simulink model "DriveTrain_Modular1"  (R2019a)
settings: Solver=FixedStepAuto  StartTime=0.0  StopTime=0.6  FixedStep=Ts  RelTol=1e-3
InitFcn:
  | DriveTrainInitialise;
undefined symbols (not defined in the file or in its folder): C, D, fsw, KdAW, KdI, KdP, KqAW, KqI, KqP, Ld, Lq, PM, Pmax, PolePairs, RotorInertia, Rs, Tmax, Ts, Tsc, Vnom
libraries: fl_lib x25, nesl_utility x13, ee_lib x5, eeGeneralControl x2, eePmsmFieldOrientedControl x1
settings Model: OrderedModelArguments=off  Creator=plewi  LastModifiedBy=plewi
settings SolverCC: ZeroCrossAlgorithm=Adaptive
settings DataIOCC: OutputOption=SpecifiedOutputTimes  OutputTimes=SDO_OutputTimes  ReturnWorkspaceOutputsName=SDOSimTest_Log
settings DebuggingCC: IgnoredZcDiagnostic=none

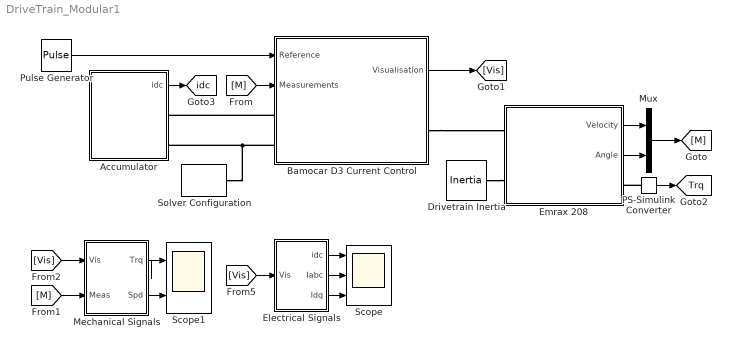
== system DriveTrain_Modular1 ==
  Accumulator : Subsystem  AncestorBlock=AccumulatorLIB/Accumulator (Simple)
  Bamocar D3 Current Control : Subsystem  AncestorBlock=InverterLIB/Bamocar D3 Current Control (Simple IGBTs)  mask(Bamocar D3 Current Controlled (Simple Diode)){Vnom=Vnom, Pmax=Pmax, Tmax=Tmax, Iq_max=800, p=PolePairs, Vdc_on=20, Ts=Ts, Tsc=Tsc, Ron=0.01, Goff=1e-8, Vf=0.5, diode_Vf=1.55, diode_Ron=0.01, diode_Goff=1e-8, RefType=Zero d-axis control, psim=PM, AxisAlignment=Q-axis, Kp_id=KdP, Ki_id=KdI, Kaw_id=KdAW, Kp_iq=KqP, Ki_iq=KqI, Kaw_iq=KqAW, AxisPrio=D-axis, CPWMMode=SVM: space vector modulation, SamplingMode=Natural, fsw=fsw}
      mask prompts: Vnom "Nominal dc-link voltage (V):"; Pmax "Maximum power (W):"; Tmax "Maximum torque (N*m):"; Iq_max "Maximum current, Iq (A):"; p "Number of rotor pole pairs:"; Vdc_on "Inverter dc-link voltage threshold (V):"; Ts "Fundamental sample time (s):"; Tsc "Control sample time (s):"; Ron "On-state resistance (Ohm):"; Goff "Off-state conductance (Siemens):"; Vf "Switching Threshold:"; diode_Vf "Forward voltage (V):"; diode_Ron "On resistance (Ohm):"; diode_Goff "Off conductance (Siemens):"; RefType "Current references:"; psim "Permanent magnet flux linkage (Wb):"; AxisAlignment "Phase-a axis alignment:"; Kp_id "D-axis current proportional gain:"; Ki_id "D-axis current integral gain:"; Kaw_id "D-axis current anti-windup gain:"; Kp_iq "Q-axis current proportional gain:"; Ki_iq "Q-axis current integral gain:"; Kaw_iq "Q-axis current anti-windup gain:"; AxisPrio "Axis prioritization:"; CPWMMode "PWM method:"; SamplingMode "Sampling mode:"; fsw "Switching frequency (Hz):"
      mask help: This block implements a PMSM field-oriented control structure, similar to the Bamocar D3. It operates under current/torque control.
      mask Help: web(nesl_help(gcbh))
      mask TypeOptions Vnom:
      | Inverter Controller/PMSM Field-Oriented
      | Control/Vnom
      mask TypeOptions Pmax:
      | Inverter Controller/PMSM Field-Oriented
      | Control/Pmax
      mask TypeOptions Tmax:
      | Inverter Controller/PMSM Field-Oriented
      | Control/Tmax
      mask TypeOptions p:
      | Inverter Controller/PMSM Field-Oriented
      | Control/p
      mask TypeOptions Vdc_on:
      | Inverter Controller/PMSM Field-Oriented
      | Control/Vdc_on
      mask TypeOptions Ts:
      | Inverter Controller/PMSM Field-Oriented
      | Control/Ts
      mask TypeOptions Tsc:
      | Inverter Controller/PMSM Field-Oriented
      | Control/Tsc
      mask TypeOptions Ron:
      | Three-Phase
      | Inverter/Switch/R_closed | Three-Phase
      | Inverter/Switch1/R_closed | Three-Phase
      | Inverter/Switch2/R_closed | Three-Phase
      | Inverter/Switch3/R_closed | Three-Phase
      | Inverter/Switch4/R_closed | Three-Phase
      | Inverter/Switch5/R_closed
      mask TypeOptions Goff:
      | Three-Phase
      | Inverter/Switch/G_open | Three-Phase
      | Inverter/Switch1/G_open | Three-Phase
      | Inverter/Switch2/G_open | Three-Phase
      | Inverter/Switch3/G_open | Three-Phase
      | Inverter/Switch4/G_open | Three-Phase
      | Inverter/Switch5/G_open
      mask TypeOptions Vf:
      | Three-Phase
      | Inverter/Switch/Threshold | Three-Phase
      | Inverter/Switch1/Threshold | Three-Phase
      | Inverter/Switch2/Threshold | Three-Phase
      | Inverter/Switch3/Threshold | Three-Phase
      | Inverter/Switch4/Threshold | Three-Phase
      | Inverter/Switch5/Threshold
      mask TypeOptions diode_Vf:
      | Three-Phase
      | Inverter/Diode1/Vf | Three-Phase
      | Inverter/Diode2/Vf | Three-Phase
      | Inverter/Diode3/Vf | Three-Phase
      | Inverter/Diode4/Vf | Three-Phase
      | Inverter/Diode5/Vf | Three-Phase
      | Inverter/Diode6/Vf
      mask TypeOptions diode_Ron:
      | Three-Phase
      | Inverter/Diode1/Ron | Three-Phase
      | Inverter/Diode2/Ron | Three-Phase
      | Inverter/Diode3/Ron | Three-Phase
      | Inverter/Diode4/Ron | Three-Phase
      | Inverter/Diode5/Ron | Three-Phase
      | Inverter/Diode6/Ron
      mask TypeOptions diode_Goff:
      | Three-Phase
      | Inverter/Diode1/Goff | Three-Phase
      | Inverter/Diode2/Goff | Three-Phase
      | Inverter/Diode3/Goff | Three-Phase
      | Inverter/Diode4/Goff | Three-Phase
      | Inverter/Diode5/Goff | Three-Phase
      | Inverter/Diode6/Goff
      mask TypeOptions RefType:
      | Inverter Controller/PMSM Field-Oriented
      | Control/RefType
      mask TypeOptions psim:
      | Inverter Controller/PMSM Field-Oriented
      | Control/psim
      mask TypeOptions AxisAlignment:
      | Inverter Controller/PMSM Field-Oriented
      | Control/AxisAlignment
      mask TypeOptions Kp_id:
      | Inverter Controller/PMSM Field-Oriented
      | Control/Kp_id
      mask TypeOptions Ki_id:
      | Inverter Controller/PMSM Field-Oriented
      | Control/Ki_id
      mask TypeOptions Kaw_id:
      | Inverter Controller/PMSM Field-Oriented
      | Control/Kaw_id
      mask TypeOptions Kp_iq:
      | Inverter Controller/PMSM Field-Oriented
      | Control/Kp_iq
      mask TypeOptions Ki_iq:
      | Inverter Controller/PMSM Field-Oriented
      | Control/Ki_iq
      mask TypeOptions Kaw_iq:
      | Inverter Controller/PMSM Field-Oriented
      | Control/Kaw_iq
      mask TypeOptions AxisPrio:
      | Inverter Controller/PMSM Field-Oriented
      | Control/AxisPrio
      mask TypeOptions CPWMMode:
      | Inverter Controller/PMSM Field-Oriented
      | Control/CPWMMode
      mask TypeOptions SamplingMode:
      | Inverter Controller/PMSM Field-Oriented
      | Control/SamplingMode
      mask TypeOptions fsw:
      | Inverter Controller/PMSM Field-Oriented
      | Control/fsw
      mask DialogControl Container4 Prompt: General
      mask DialogControl Container11 Prompt: Electrical
      mask DialogControl Container12 Prompt: Capacitor Bank
      mask DialogControl Container16 Prompt: IGBTs
      mask DialogControl Container17 Prompt: Protection Diodes
      mask DialogControl Container5 Prompt: Outer Loop
      mask DialogControl Container6 Prompt: Inner Loop
      mask DialogControl Container7 Prompt: PWM
      mask Display: image('C:\Users\plewi\Documents\University\6-Sixth Year\MUR\MUR-E_Simulation_2019\Images\bamocar_d3.PNG');
  Drivetrain Inertia : fl_lib/Mechanical/Rotational Elements/Inertia  inertia=J kg*m^2  w_specify=off  w_priority=High  w=0 rad/s  w_nominal_specify=off  w_nominal_unit=rad/s  w_nominal_value=1  t_specify=off  t_priority=None  t=0 N*m  t_nominal_specify=off  t_nominal_unit=N*m  t_nominal_value=1
  Electrical Signals : Subsystem
  Emrax 208 : Subsystem  AncestorBlock=MotorLIB/Emrax 208  mask(Emrax 208){nPolePairs=PolePairs, pm_flux_linkage=PM, Ld=Ld, Lq=Lq, L0=0, Rs=Rs, zero_sequence=ee.enum.park.zerosequence.exclude, J=RotorInertia}
      mask prompts: nPolePairs "Number of pole pairs"; pm_flux_linkage "Permanent magnet flux linkage"; Ld "Stator d-axis inductance, Ld"; Lq "Stator q-axis inductance, Lq"; L0 "Stator zero-sequence inductance, L0"; Rs "Stator resistance per phase, Rs"; zero_sequence "Zero sequence"; J "Rotor inertia (g cm^2)"
      mask TypeOptions nPolePairs:
      | Permanent Magnet
      | Synchronous Motor/nPolePairs
      mask TypeOptions pm_flux_linkage:
      | Permanent Magnet
      | Synchronous Motor/pm_flux_linkage
      mask TypeOptions Ld:
      | Permanent Magnet
      | Synchronous Motor/Ld
      mask TypeOptions Lq:
      | Permanent Magnet
      | Synchronous Motor/Lq
      mask TypeOptions L0:
      | Permanent Magnet
      | Synchronous Motor/L0
      mask TypeOptions Rs:
      | Permanent Magnet
      | Synchronous Motor/Rs
      mask TypeOptions zero_sequence:
      | Permanent Magnet
      | Synchronous Motor/zero_sequence
      mask TypeOptions J:
      | Permanent Magnet
      | Synchronous Motor/J
      mask DialogControl Container4 Prompt: Main
  Mechanical Signals : Subsystem
  Mux : Mux  Inputs=2
  PS-Simulink Converter : nesl_utility/PS-Simulink Converter  PhysicalDomain=network_engine_domain  SubClassName=ps_output  LeftPortType=input  RightPortType=output  PseudoPeriodic=off  Frequencies=[]  Unit=1  AffineConversion=off
  Pulse Generator : DiscretePulseGenerator  PulseType=Time based  Amplitude=5  Period=0.6  PulseWidth=50  PhaseDelay=0.05
  Scope : Scope  NumInputPorts=3
  Scope1 : Scope  NumInputPorts=2
  Solver Configuration : nesl_utility/Solver Configuration  PhysicalDomain=network_engine_domain  SubClassName=solver  LeftPortType=input  RightPortType=generic  Tones=[]  Harmonics=[]  SimulateNoise=off  Profile=off  UseLocalSampling=off  EnableSwitchedLinearOptims=on  FrequencyDomain=off  UseCCode=off  RelTol=0.001  AbsTol=1e-06  MinStep=1e-09  ToWorkspace=off  RevertToSquareIcSolve=off  NumHomotopyIterations=100  PhasorMode=off  PhasorModeNumHarmonics=1  DoDC=off  ResidualTolerance=1e-09  UseLocalSolver=off  LocalSolverChoice=NE_BACKWARD_EULER_ADVANCER  LocalSolverSampleTime=0.001  DoFixedCost=off  MaxNonlinIter=3  MaxModeIter=2  LinearAlgebra=auto  EquationFormulation=NE_TIME_EF  DelaysMemoryBudget=1024  AutomaticFiltering=on  FilteringTimeConstant=0.001  PartitionStorageMethod=AS_NEEDED  PartitionMemoryBudget=1024  PartitionMethod=ROBUST
  tag scope: Trq=global, idc=global
  wires:
  Mux/1 -> [M]
  [M] -> Bamocar D3 Current Control/2(Measurements)
  Emrax 208/1(Velocity) -> Mux/1
  Emrax 208/2(Angle) -> Mux/2
  Bamocar D3 Current Control/1(Visualisation) -> [Vis]
  PS-Simulink Converter/1 -> [Trq]
  Accumulator/1(idc) -> [idc]
  Electrical Signals/1(idc) -> Scope/1
  Electrical Signals/3(Idq) -> Scope/3
  [M] -> Mechanical Signals/2("Meas ")
  [Vis] -> Mechanical Signals/1(Vis)
  Electrical Signals/2(Iabc) -> Scope/2
  Mechanical Signals/1(Trq) -> Scope1/1
  Mechanical Signals/2(Spd) -> Scope1/2
  [Vis] -> Electrical Signals/1(Vis)
  Pulse Generator/1 -> Bamocar D3 Current Control/1(Reference)
  connections:
  Bamocar D3 Current Control/LConn2 -- Solver Configuration/RConn1 -- Accumulator/RConn2
  PS-Simulink Converter/LConn1 -- Emrax 208/RConn1
  Bamocar D3 Current Control/LConn1 -- Accumulator/RConn1
  Bamocar D3 Current Control/RConn1 -- Emrax 208/LConn1
  Drivetrain Inertia/LConn1 -- Emrax 208/LConn2

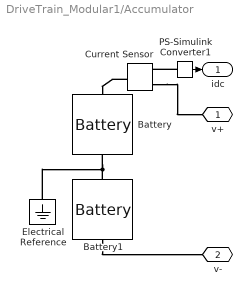
== system DriveTrain_Modular1/Accumulator ==
  Battery : ee_lib/Sources/Battery  Vnom=Vnom/2 V  R1=0.001 Ohm  prm_AH=1  AH=14000 hr*A  V1=470 V  AH1=5000 hr*A  prm_R2=1  R2=inf Ohm  prm_dyn=1  Rp1=0.005 Ohm  tau1=30 s  Rp2=0.005 Ohm  tau2=30 s  Rp3=0.005 Ohm  tau3=30 s  Rp4=0.005 Ohm  tau4=30 s  Rp5=0.005 Ohm  tau5=30 s  prm_fade=1  N_fade=100  AH_fade=45 hr*A  R1_fade=2.02 Ohm  V1_fade=10.35 V  i_specify=off  i_priority=Low  i=0 A  i_nominal_specify=off  i_nominal_unit=A  i_nominal_value=1  v_specify=on  v_priority=High  v=Vnom/2 V  v_nominal_specify=off  v_nominal_unit=V  v_nominal_value=1  charge_specify=on  charge_priority=None  charge=7000 hr*A  charge_nominal_specify=off  charge_nominal_unit=hr*A  charge_nominal_value=1  num_cycles_specify=on  num_cycles_priority=None  num_cycles=0  num_cycles_nominal_specify=off  num_cycles_nominal_unit=1  num_cycles_nominal_value=1  thermal_mass=30000 J/K  Tmeas=298.15 K  Vnom_T2=12 V  R1_T2=2.2 Ohm  V1_T2=11.4 V  R2_T2=2200 Ohm  Rp1_T2=0.005 Ohm  tau1_T2=30 s  Rp2_T2=0.005 Ohm  tau2_T2=30 s  Rp3_T2=0.005 Ohm  tau3_T2=30 s  Rp4_T2=0.005 Ohm  tau4_T2=30 s  Rp5_T2=0.005 Ohm  tau5_T2=30 s  Tmeas2=273.15 K  temperature_specify=off  temperature_priority=High  temperature=298.15 K  temperature_nominal_specify=off  temperature_nominal_unit=K  temperature_nominal_value=1
      settings: SourceProductName=Simscape Electrical
  Battery1 : ee_lib/Sources/Battery  Vnom=Vnom/2 V  R1=0.001 Ohm  prm_AH=1  AH=14000 hr*A  V1=470 V  AH1=5000 hr*A  prm_R2=1  R2=inf Ohm  prm_dyn=1  Rp1=0.005 Ohm  tau1=30 s  Rp2=0.005 Ohm  tau2=30 s  Rp3=0.005 Ohm  tau3=30 s  Rp4=0.005 Ohm  tau4=30 s  Rp5=0.005 Ohm  tau5=30 s  prm_fade=1  N_fade=100  AH_fade=45 hr*A  R1_fade=2.02 Ohm  V1_fade=10.35 V  i_specify=off  i_priority=Low  i=0 A  i_nominal_specify=off  i_nominal_unit=A  i_nominal_value=1  v_specify=on  v_priority=High  v=Vnom/2 V  v_nominal_specify=off  v_nominal_unit=V  v_nominal_value=1  charge_specify=on  charge_priority=None  charge=7000 hr*A  charge_nominal_specify=off  charge_nominal_unit=hr*A  charge_nominal_value=1  num_cycles_specify=on  num_cycles_priority=None  num_cycles=0  num_cycles_nominal_specify=off  num_cycles_nominal_unit=1  num_cycles_nominal_value=1  thermal_mass=30000 J/K  Tmeas=298.15 K  Vnom_T2=12 V  R1_T2=2.2 Ohm  V1_T2=11.4 V  R2_T2=2200 Ohm  Rp1_T2=0.005 Ohm  tau1_T2=30 s  Rp2_T2=0.005 Ohm  tau2_T2=30 s  Rp3_T2=0.005 Ohm  tau3_T2=30 s  Rp4_T2=0.005 Ohm  tau4_T2=30 s  Rp5_T2=0.005 Ohm  tau5_T2=30 s  Tmeas2=273.15 K  temperature_specify=off  temperature_priority=High  temperature=298.15 K  temperature_nominal_specify=off  temperature_nominal_unit=K  temperature_nominal_value=1
      settings: SourceProductName=Simscape Electrical
  Current Sensor : fl_lib/Electrical/Electrical Sensors/Current Sensor
  Electrical Reference : fl_lib/Electrical/Electrical Elements/Electrical Reference
      settings: SourceProductName=Foundation Library
  PS-Simulink Converter1 : nesl_utility/PS-Simulink Converter  PhysicalDomain=network_engine_domain  SubClassName=ps_output  LeftPortType=input  RightPortType=output  PseudoPeriodic=off  Frequencies=[]  Unit=1  AffineConversion=off
  v+ : PMIOPort  Side=Right
  v- : PMIOPort  Port=2  Side=Right
  idc : Outport
  wires:
  PS-Simulink Converter1/1 -> idc/1
  connections:
  Battery1/RConn1 -- v-/RConn1
  PS-Simulink Converter1/LConn1 -- Current Sensor/RConn1
  Current Sensor/RConn2 -- v+/RConn1
  Current Sensor/LConn1 -- Battery/LConn1
  Battery1/LConn1 -- Electrical Reference/LConn1 -- Battery/RConn1

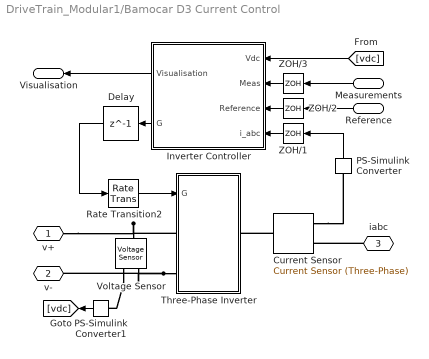
== system DriveTrain_Modular1/Bamocar D3 Current Control ==
  Reference : Inport
  Measurements : Inport  Port=2
  Current Sensor : ee_lib/Sensors & Transducers/Current Sensor (Three-Phase)
      settings: SourceProductName=Simscape Electrical
  Delay : Delay  DelayLength=1
  Inverter Controller : Subsystem
  PS-Simulink Converter : nesl_utility/PS-Simulink Converter  PhysicalDomain=network_engine_domain  SubClassName=ps_output  LeftPortType=input  RightPortType=output  PseudoPeriodic=off  Frequencies=[]  Unit=1  AffineConversion=off
  PS-Simulink Converter1 : nesl_utility/PS-Simulink Converter  PhysicalDomain=network_engine_domain  SubClassName=ps_output  LeftPortType=input  RightPortType=output  PseudoPeriodic=off  Frequencies=[]  Unit=1  AffineConversion=off
  Rate Transition2 : RateTransition  OutPortSampleTime=Ts
  Three-Phase Inverter : Subsystem
  Voltage Sensor : fl_lib/Electrical/Electrical Sensors/Voltage Sensor
  ZOH/1 : ZeroOrderHold  SampleTime=Tsc
  ZOH/2 : ZeroOrderHold  SampleTime=Tsc
  ZOH/3 : ZeroOrderHold  SampleTime=Tsc
  v+ : PMIOPort  Side=Left
  v- : PMIOPort  Port=2  Side=Left
  iabc : PMIOPort  Port=3  Side=Right
  Visualisation : Outport
  wires:
  Measurements/1 -> ZOH/3/1
  Delay/1 -> Rate Transition2/1
  Inverter Controller/2(G) -> Delay/1
  ZOH/1/1 -> Inverter Controller/4(i_abc)
  PS-Simulink Converter/1 -> ZOH/1/1
  ZOH/2/1 -> Inverter Controller/3(Reference)
  Rate Transition2/1 -> Three-Phase Inverter/1(G)
  Inverter Controller/1(Visualisation) -> Visualisation/1
  PS-Simulink Converter1/1 -> [vdc]
  [vdc] -> Inverter Controller/1(Vdc)
  ZOH/3/1 -> Inverter Controller/2(Meas)
  Reference/1 -> ZOH/2/1
  connections:
  Voltage Sensor/LConn1 -- v+/RConn1 -- Three-Phase Inverter/LConn1
  Three-Phase Inverter/LConn2 -- v-/RConn1 -- Voltage Sensor/RConn2
  Current Sensor/LConn1 -- Three-Phase Inverter/RConn1
  Current Sensor/RConn1 -- PS-Simulink Converter/LConn1
  Voltage Sensor/RConn1 -- PS-Simulink Converter1/LConn1
  iabc/RConn1 -- Current Sensor/RConn2

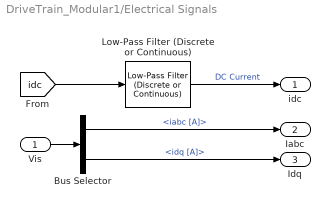
== system DriveTrain_Modular1/Electrical Signals ==
  Vis : Inport
  Bus Selector : BusSelector  OutputSignals=signal2.iabc [A],signal2.idq [A]
  Low-Pass Filter (Discrete or Continuous) : eeGeneralControl/Low-Pass Filter (Discrete or Continuous)  K=1  T=4e-3  B=inf  A=-inf  Ts=-1
      settings: SourceProductName=Simscape Electrical
  idc : Outport
  Iabc : Outport  Port=2
  Idq : Outport  Port=3
  wires:
  Low-Pass Filter (Discrete or Continuous)/1 -> idc/1  "DC Current"
  [idc] -> Low-Pass Filter (Discrete or Continuous)/1
  Vis/1 -> Bus Selector/1
  Bus Selector/1 -> Iabc/1  "<iabc [A]>"
  Bus Selector/2 -> Idq/1  "<idq [A]>"

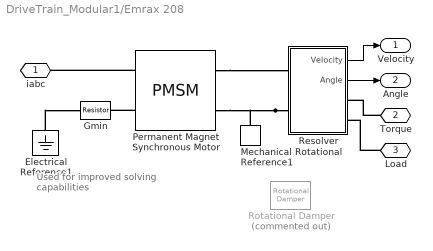
== system DriveTrain_Modular1/Emrax 208 ==
  note: Used for improved
      | solving capabilities
  Electrical Reference1 : fl_lib/Electrical/Electrical Elements/Electrical Reference
  Gmin : fl_lib/Electrical/Electrical Elements/Resistor  R=1e9 Ohm  i_specify=off  i_priority=High  i=0 A  i_nominal_specify=off  i_nominal_unit=A  i_nominal_value=1  v_specify=off  v_priority=High  v=0 V  v_nominal_specify=off  v_nominal_unit=V  v_nominal_value=1
  Mechanical Rotational Reference1 : fl_lib/Mechanical/Rotational Elements/Mechanical Rotational Reference
  Permanent Magnet Synchronous Motor : ee_lib/Electromechanical/Permanent Magnet/PMSM  nPolePairs=nPolePairs  pmflux_param=1  pm_flux_linkage=pm_flux_linkage Wb  torque_constant=0.18 N*m/A  back_emf_constant=0.18 V/(rad/s)  stator_param=1  Ld=Ld H  Lq=Lq H  L0=L0 H  Ls=0.0002 H  Lm=0.00002 H  Ms=0.00002 H  Rs=Rs Ohm  zero_sequence=zero_sequence  J=J g*cm^2  lam=0.01 N*m/(rad/s)  axes_param=ee.enum.rotorangle.qaxis  i_d_specify=off  i_d_priority=None  i_d=0 A  i_d_nominal_specify=off  i_d_nominal_unit=A  i_d_nominal_value=1  i_q_specify=off  i_q_priority=None  i_q=0 A  i_q_nominal_specify=off  i_q_nominal_unit=A  i_q_nominal_value=1  torque_specify=off  torque_priority=None  torque=0 N*m  torque_nominal_specify=off  torque_nominal_unit=N*m  torque_nominal_value=1  angular_velocity_specify=on  angular_velocity_priority=High  angular_velocity=0 rpm  angular_velocity_nominal_specify=off  angular_velocity_nominal_unit=rpm  angular_velocity_nominal_value=1  angular_position_specify=on  angular_position_priority=High  angular_position=0 rad  angular_position_nominal_specify=off  angular_position_nominal_unit=deg  angular_position_nominal_value=1
      settings: SourceProductName=Simscape Electrical
  Resolver : Subsystem
  Rotational Damper : fl_lib/Mechanical/Rotational Elements/Rotational Damper  Commented=on  D=D N*m/(rad/s)  w_specify=off  w_priority=None  w=0 rad/s  w_nominal_specify=off  w_nominal_unit=rad/s  w_nominal_value=1  t_specify=off  t_priority=None  t=0 N*m  t_nominal_specify=off  t_nominal_unit=N*m  t_nominal_value=1
  iabc : PMIOPort  Side=Left
  Torque : PMIOPort  Port=2  Side=Right
  Load : PMIOPort  Port=3  Side=Left
  Velocity : Outport
  Angle : Outport  Port=2
  wires:
  Resolver/2(Angle) -> Angle/1
  Resolver/1(Velocity) -> Velocity/1
  connections:
  Torque/RConn1 -- Resolver/RConn1
  Permanent Magnet Synchronous Motor/LConn1 -- iabc/RConn1
  Permanent Magnet Synchronous Motor/LConn2 -- Gmin/RConn1
  Load/RConn1 -- Resolver/RConn2
  Resolver/LConn2 -- Permanent Magnet Synchronous Motor/RConn2 -- Mechanical Rotational Reference1/LConn1
  Electrical Reference1/LConn1 -- Gmin/LConn1
  Permanent Magnet Synchronous Motor/RConn1 -- Resolver/LConn1

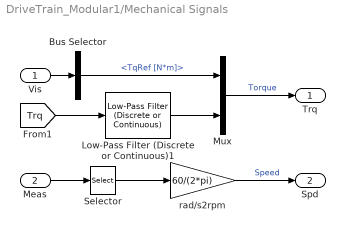
== system DriveTrain_Modular1/Mechanical Signals ==
  Vis : Inport
  "Meas " : Inport  Port=2
  Bus Selector : BusSelector  OutputSignals=signal2.TqRef [N*m]
  Low-Pass Filter (Discrete or Continuous)1 : eeGeneralControl/Low-Pass Filter (Discrete or Continuous)  K=1  T=4e-2  B=inf  A=-inf  Ts=-1
      settings: SourceProductName=Simscape Electrical
  Mux : Mux  Inputs=2
  Selector : Selector  InputPortWidth=2  IndexOptions=Index vector (dialog)  Indices=[1]  OutputSizes=1
  rad/s2rpm : Gain  Gain=60/(2*pi)
  Trq : Outport
  Spd : Outport  Port=2
  wires:
  Vis/1 -> Bus Selector/1
  rad/s2rpm/1 -> Spd/1  "Speed"
  Selector/1 -> rad/s2rpm/1
  Mux/1 -> Trq/1  "Torque"
  Bus Selector/1 -> Mux/1  "<TqRef [N*m]>"
  "Meas "/1 -> Selector/1
  [Trq] -> Low-Pass Filter (Discrete or Continuous)1/1
  Low-Pass Filter (Discrete or Continuous)1/1 -> Mux/2

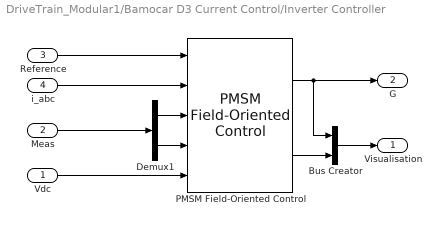
== system DriveTrain_Modular1/Bamocar D3 Current Control/Inverter Controller ==
  Vdc : Inport
  Meas : Inport  Port=2
  Reference : Inport  Port=3
  i_abc : Inport  Port=4
  Bus Creator : BusCreator  Inputs=2
  Demux1 : Demux  Outputs=2
  PMSM Field-Oriented Control : eePmsmFieldOrientedControl/PMSM Field-Oriented Control  CtrlMode=Torque control  Vnom=Vnom  Pmax=Pmax  Tmax=Tmax  p=p  Vdc_on=Vdc_on  Ts=Ts  Tsc=Tsc  CtrlType=PI control  Kp_w=50  Ki_w=500  Kv_w=1  Kaw_w=1000  RefType=Zero d-axis control  rpmVec=[0, 3000]  TqVec=[-100, 0, 100]  VdcVec=[300, 350]  idMatrix=zeros(2,3,2)  iqMatrix=zeros(2,3,2)  psim=psim  Ld=0.00024  Lq=0.00029  Rs=0.01  AxisAlignment=Q-axis  Kp_id=Kp_id  Ki_id=Ki_id  Kaw_id=Kaw_id  Kp_iq=Kp_iq  Ki_iq=Ki_iq  Kaw_iq=Kaw_iq  AxisPrio=D-axis  ActZC=on  ActFF=off  ParamTypeFF=Constant parameters  LdFF=Ld  LqFF=Lq  psimFF=PM  idVect=[-200, 0, 200]  iqVect=[-200, 0, 200]  LdMatrix=0.0002 * ones(3, 3)  LqMatrix=0.0002 * ones(3, 3)  psimMatrix=0.04 * ones(3, 3)  CPWMMode=SVM: space vector modulation  fsw=fsw
      settings: SourceProductName=Simscape Electrical  SourceProductBaseCode=PS
  Visualisation : Outport
  G : Outport  Port=2
  wires:
  Bus Creator/1 -> Visualisation/1
  PMSM Field-Oriented Control/2 -> Bus Creator/2
  PMSM Field-Oriented Control/1 -> G/1, Bus Creator/1
  Vdc/1 -> PMSM Field-Oriented Control/5
  i_abc/1 -> PMSM Field-Oriented Control/2
  Meas/1 -> Demux1/1
  Demux1/1 -> PMSM Field-Oriented Control/3
  Demux1/2 -> PMSM Field-Oriented Control/4
  Reference/1 -> PMSM Field-Oriented Control/1

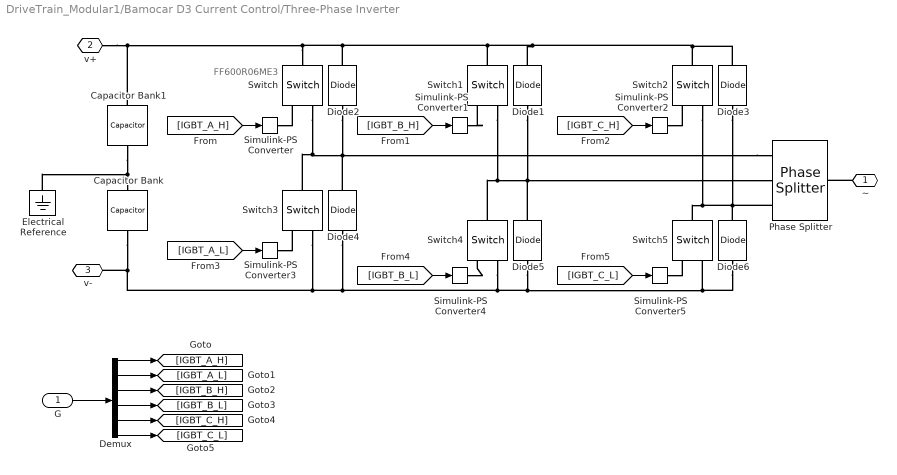
== system DriveTrain_Modular1/Bamocar D3 Current Control/Three-Phase Inverter ==
  note: FF600R06ME3
  G : Inport
  Capacitor Bank : fl_lib/Electrical/Electrical Elements/Capacitor  c=C/2 uF  r=0 Ohm  g=0 1/Ohm  i_specify=off  i_priority=None  i=0 A  i_nominal_specify=off  i_nominal_unit=A  i_nominal_value=1  v_specify=off  v_priority=None  v=0 V  v_nominal_specify=off  v_nominal_unit=V  v_nominal_value=1  vc_specify=on  vc_priority=High  vc=Vnom/2 V  vc_nominal_specify=off  vc_nominal_unit=V  vc_nominal_value=1
  Capacitor Bank1 : fl_lib/Electrical/Electrical Elements/Capacitor  c=C/2 uF  r=0 Ohm  g=0 1/Ohm  i_specify=off  i_priority=None  i=0 A  i_nominal_specify=off  i_nominal_unit=A  i_nominal_value=1  v_specify=off  v_priority=None  v=0 V  v_nominal_specify=off  v_nominal_unit=V  v_nominal_value=1  vc_specify=on  vc_priority=None  vc=Vnom/2 V  vc_nominal_specify=off  vc_nominal_unit=V  vc_nominal_value=1
  Demux : Demux  Outputs=6
  Diode{1..6} (6 alike) : fl_lib/Electrical/Electrical Elements/Diode  Vf=diode_Vf V  Ron=diode_Ron Ohm  Goff=diode_Goff 1/Ohm  i_specify=off  i_priority=None  i=0 A  i_nominal_specify=off  i_nominal_unit=A  i_nominal_value=1  v_specify=off  v_priority=None  v=0 V  v_nominal_specify=off  v_nominal_unit=V  v_nominal_value=1
  Electrical Reference : fl_lib/Electrical/Electrical Elements/Electrical Reference
      settings: SourceProductName=Foundation Library
  Phase Splitter : ee_lib/Connectors & References/Phase Splitter
      settings: SourceProductName=Simscape Electrical  SourceProductBaseCode=PS
  Simulink-PS Converter{,1..5} (6 alike) : nesl_utility/Simulink-PS Converter  PhysicalDomain=network_engine_domain  SubClassName=ps_input  LeftPortType=input  RightPortType=output  PseudoPeriodic=off  Frequencies=[]  NoiseDistribution=none  NoiseParameters=[]  Unit=1  AffineConversion=off  FilteringAndDerivatives=provide  SimscapeFilterOrder=1  InputFilterTimeConstant=0.001  UdotUserProvided=0
  Switch{,1..5} (6 alike) : fl_lib/Electrical/Electrical Elements/Switch  R_closed=Ron Ohm  G_open=Goff 1/Ohm  Threshold=Vf  i_specify=off  i_priority=None  i=0 A  i_nominal_specify=off  i_nominal_unit=A  i_nominal_value=1  v_specify=off  v_priority=None  v=0 V  v_nominal_specify=off  v_nominal_unit=V  v_nominal_value=1
      settings: SourceProductName=Simscape
  ~ : PMIOPort  Tag=PMCPort  Side=Right
  v+ : PMIOPort  Tag=PMCPort  Port=2  Side=Left
  v- : PMIOPort  Tag=PMCPort  Port=3  Side=Left
  wires:
  Demux/6 -> [IGBT_C_L]
  Demux/5 -> [IGBT_C_H]
  Demux/4 -> [IGBT_B_L]
  Demux/3 -> [IGBT_B_H]
  Demux/2 -> [IGBT_A_L]
  Demux/1 -> [IGBT_A_H]
  [IGBT_C_L] -> Simulink-PS Converter5/1
  [IGBT_B_L] -> Simulink-PS Converter4/1
  [IGBT_A_L] -> Simulink-PS Converter3/1
  [IGBT_C_H] -> Simulink-PS Converter2/1
  [IGBT_B_H] -> Simulink-PS Converter1/1
  [IGBT_A_H] -> Simulink-PS Converter/1
  G/1 -> Demux/1
  connections:
  Capacitor Bank1/RConn1 -- Electrical Reference/LConn1 -- Capacitor Bank/LConn1
  Switch5/LConn1 -- Switch2/RConn2 -- Diode6/RConn1 -- Diode3/LConn1 -- Phase Splitter/RConn3
  Diode5/RConn1 -- Diode1/LConn1 -- Phase Splitter/RConn2 -- Switch1/RConn2 -- Switch4/LConn1
  Simulink-PS Converter5/RConn1 -- Switch5/RConn1
  Simulink-PS Converter4/RConn1 -- Switch4/RConn1
  Simulink-PS Converter3/RConn1 -- Switch3/RConn1
  Simulink-PS Converter2/RConn1 -- Switch2/RConn1
  Simulink-PS Converter1/RConn1 -- Switch1/RConn1
  Simulink-PS Converter/RConn1 -- Switch/RConn1
  Switch/LConn1 -- Diode2/RConn1 -- Switch1/LConn1 -- Diode3/RConn1 -- Switch2/LConn1 -- Diode1/RConn1 -- Capacitor Bank1/LConn1 -- v+/RConn1
  v-/RConn1 -- Switch4/RConn2 -- Diode5/LConn1 -- Switch5/RConn2 -- Diode6/LConn1 -- Diode4/LConn1 -- Switch3/RConn2 -- Capacitor Bank/RConn1
  Phase Splitter/RConn1 -- Diode2/LConn1 -- Diode4/RConn1 -- Switch3/LConn1 -- Switch/RConn2
  ~/RConn1 -- Phase Splitter/LConn1

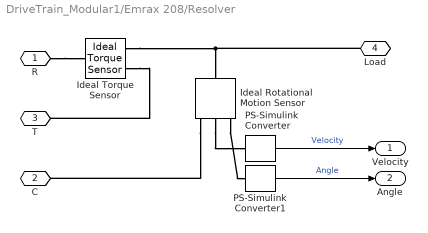
== system DriveTrain_Modular1/Emrax 208/Resolver ==
  Ideal Rotational Motion Sensor : fl_lib/Mechanical/Mechanical Sensors/Ideal Rotational Motion Sensor  offset=0 deg
      settings: SourceProductName=Foundation Library
  Ideal Torque Sensor : fl_lib/Mechanical/Mechanical Sensors/Ideal Torque Sensor
      settings: SourceProductName=Foundation Library
  PS-Simulink Converter : nesl_utility/PS-Simulink Converter  PhysicalDomain=network_engine_domain  SubClassName=ps_output  LeftPortType=input  RightPortType=output  PseudoPeriodic=off  Frequencies=[]  Unit=rad/s  AffineConversion=off
  PS-Simulink Converter1 : nesl_utility/PS-Simulink Converter  PhysicalDomain=network_engine_domain  SubClassName=ps_output  LeftPortType=input  RightPortType=output  PseudoPeriodic=off  Frequencies=[]  Unit=rad  AffineConversion=off
  R : PMIOPort  Side=Left
  C : PMIOPort  Port=2  Side=Left
  T : PMIOPort  Port=3  Side=Right
  Load : PMIOPort  Port=4  Side=Right
  Velocity : Outport
  Angle : Outport  Port=2
  wires:
  PS-Simulink Converter/1 -> Velocity/1  "Velocity"
  PS-Simulink Converter1/1 -> Angle/1  "Angle"
  connections:
  Ideal Rotational Motion Sensor/RConn3 -- PS-Simulink Converter1/LConn1
  Ideal Rotational Motion Sensor/RConn2 -- PS-Simulink Converter/LConn1
  Ideal Torque Sensor/RConn1 -- Load/RConn1 -- Ideal Rotational Motion Sensor/LConn1
  Ideal Rotational Motion Sensor/RConn1 -- C/RConn1
  R/RConn1 -- Ideal Torque Sensor/LConn1
  Ideal Torque Sensor/RConn2 -- T/RConn1
